simulink model "PMRAC_non_time_delay_final"  (R2022a)
settings: Solver=ode45  StartTime=0.0  StopTime=50  RelTol=1e-3  EnableMultiTasking=on
settings Model: Creator=Administrator  LastModifiedBy=mluser
settings SolverCC: AlgebraicLoopSolver=TrustRegion
settings DataIOCC: LimitDataPoints=on  SaveFormat=Array  ReturnWorkspaceOutputs=off
settings OptimizationCC: LifeSpan=inf
settings DebuggingCC: SolverPrmCheckMsg=warning  UnconnectedInputMsg=warning  UnconnectedOutputMsg=warning  UnconnectedLineMsg=warning  AllowSymbolicDim=off  SFUnexpectedBacktrackingDiag=warning  SFNoUnconditionalDefaultTransitionDiag=warning  SFExecutionAtInitializationDiag=none  SFMachineParentedDataDiag=warning  ArithmeticOperatorsInVariantConditions=warning
settings HardwareCC: ProdBitPerPointer=32  ProdBitPerSizeT=32  ProdBitPerPtrDiffT=32  ProdLargestAtomicFloat=None  ProdIntDivRoundTo=Undefined  ProdEndianess=Unspecified  ProdWordSize=32  ProdHWDeviceType=32-bit Generic
settings ModelReferenceCC: PropagateSignalLabelsOutOfModel=off
settings SFSimCC: SimUseLocalCustomCode=off  CustomCodeUndefinedFunction=UseInterfaceOnly
settings RTWCC: RTWUseLocalCustomCode=off
settings CodeAppCC: StateflowObjectComments=on
settings GRTTargetCC: TargetLangStandard=C89/C90 (ANSI)
settings ConfigComp: CovMetricSettings=dw  CovSaveCumulativeToWorkspaceVar=on  CovSaveSingleToWorkspaceVar=on  CovExternalEMLEnable=off  CovSFcnEnable=off

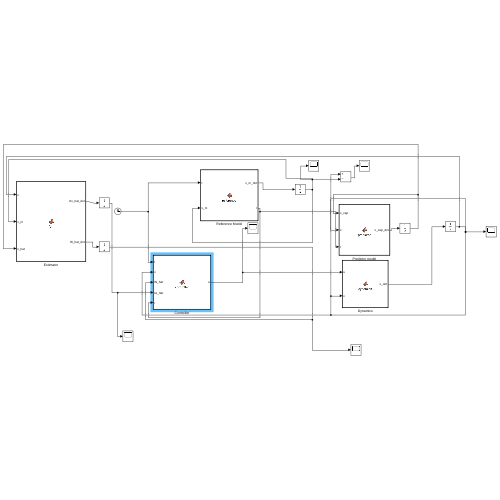
[thumbnail: Simulink's stored preview of the top-level diagram]
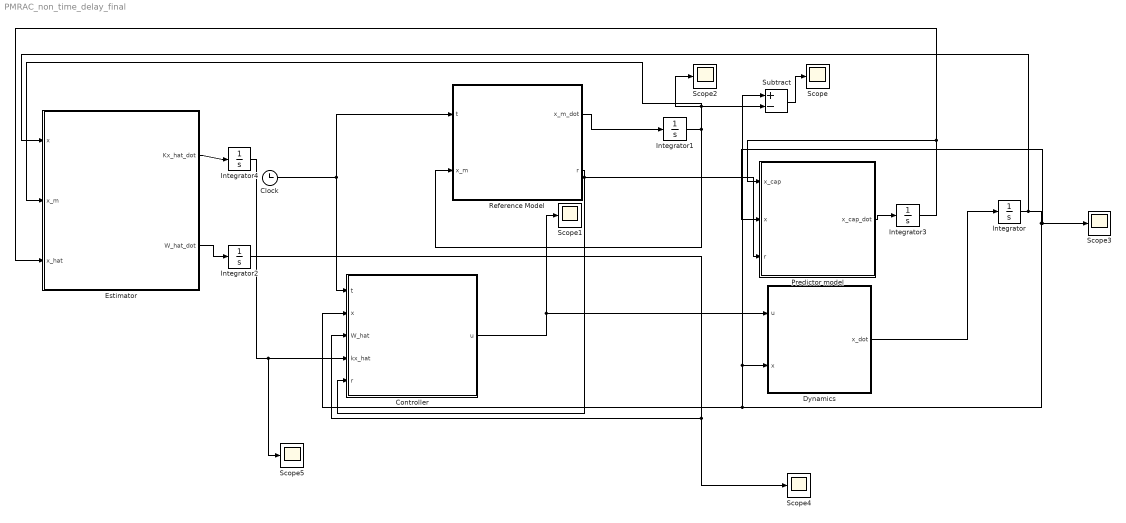
== system PMRAC_non_time_delay_final ==
  Clock : Clock
      settings: Decimation=50
  Controller : MATLAB Function  TreatAsAtomicUnit=on
  Dynamics : MATLAB Function  TreatAsAtomicUnit=on
  Estimator : MATLAB Function  TreatAsAtomicUnit=on
  Integrator : Integrator  InitialCondition=[-1;1]
  Integrator1 : Integrator  InitialCondition=[0;0]
  Integrator2 : Integrator  InitialCondition=zeros(6,1)
  Integrator3 : Integrator  InitialCondition=[-1;1]
  Integrator4 : Integrator  InitialCondition=zeros(2,1)
  Predictor model : MATLAB Function  TreatAsAtomicUnit=on
  Reference Model : MATLAB Function  TreatAsAtomicUnit=on
  Scope{,1..5} (6 alike) : Scope
  Subtract : Sum  Inputs=+-
  wires:
  Dynamics/1(x_dot) -> Integrator/1
  Integrator/1 -> Estimator/1(x), Predictor model/2(x), Scope3/1, Subtract/1, Dynamics/2(x), Controller/2(x)
  Clock/1 -> Controller/1(t), Reference Model/1(t)
  Controller/1(u) -> Scope1/1, Dynamics/1(u)
  Reference Model/1(x_m_dot) -> Integrator1/1
  Integrator1/1 -> Estimator/2(x_m), Subtract/2, Scope2/1, Reference Model/2(x_m)
  Integrator2/1 -> Scope4/1, Controller/3(W_hat)
  Subtract/1 -> Scope/1
  Predictor model/1(x_cap_dot) -> Integrator3/1
  Integrator3/1 -> Estimator/3(x_hat), Predictor model/1(x_cap)
  Estimator/2(W_hat_dot) -> Integrator2/1
  Estimator/1(Kx_hat_dot) -> Integrator4/1
  Integrator4/1 -> Scope5/1, Controller/4(kx_hat)
  Reference Model/2(r) -> Controller/5(r), Predictor model/3(r)

== matlab function PMRAC_non_time_delay_final/Controller ==
  data: u output; t input; x input; W_hat input; kx_hat input; r input
function u   = controller(t,x,W_hat,kx_hat,r)

%r=10;
%r=exp(-t);

%r=2*sin(t);

%k_x=[-2/3 -1/3]'; % note that the linear control gain is directly chosen instead of adapting with an assumption of $A$ matrix to be known
theta=x(1,1);
p=x(2,1);
phi_bar = [1; theta; p; abs(theta)*p; abs(p)*p; theta^3];

u=kx_hat'*x+r-W_hat'*phi_bar;

end

== matlab function PMRAC_non_time_delay_final/Dynamics ==
  data: u input; x input; x_dot output
function x_dot    = dynamics(u,x)

L_delta_a=1;

A=[0 1; 0 0];

a0=0.8;
a1=0.2314;
a2=0.6918;
a3=-0.6245;
a4=0.0095;
a5=0.0214;

B=[0 1]';

theta=x(1,1);
p=x(2,1);

%W = [a0;a1;a2;a3;a4;a5];
%phi_bar = [1; theta; p; abs(theta)*p; abs(p)*p; theta^3];
%phi_bar =[1;1;1;1;1;1];

delta=a0+a1*theta+a2*p+a3*abs(theta)*p+a4*abs(p)*p+a5*theta^3;
x_dot=A*x+B*(u+delta/L_delta_a);
end

== matlab function PMRAC_non_time_delay_final/Predictor model ==
  data: x_cap_dot output; x_cap input; x input; r input
function x_cap_dot = predictor( x_cap, x, r)


am1=-2;
am2=-1;
A_ref=[0 1; am1 am2];

A_prd =4* A_ref;


L_delta_a=1;
B_c=[0; L_delta_a];

x_cap_dot = A_prd*(x_cap-x) + A_ref*x + B_c*r;

== matlab function PMRAC_non_time_delay_final/Reference Model ==
  data: x_m_dot output; t input; x_m input; r output
function [x_m_dot,r]  = reference(t,x_m)
am1=-2;
am2=-1;
L_delta_a=1;
%r=exp(-t);
r=sin(t);
%r=2*sin(t);
%A_ref=A+B*k_x';
A_ref=[0 1; am1 am2];
B_c=[0; L_delta_a];
x_m_dot=A_ref*x_m+B_c*r;

== matlab function PMRAC_non_time_delay_final/Estimator ==
  data: Kx_hat_dot output; W_hat_dot output; x input; x_m input; x_hat input
function [Kx_hat_dot, W_hat_dot] = fcn(x, x_m, x_hat)

%gamma_x = [1,0;
 %          2,1];
gamma_x=2*eye(2);
%gamma_w = [1,0,1,2,3,4;
  %         3,4,1,2,5,6;
  %         5,2,1,6,8,3;
  %         2,4,5,7,2,1;
  %         4,5,1,2,6,3;
  %         7,9,0,1,3,0];
gamma_w=100*eye(6);

theta=x(1,1);
p=x(2,1);
phi_bar = [1; theta; p; abs(theta)*p; abs(p)*p; theta^3];

%P_ref = [1.75,-0.5;-0.5,3];
%P_ref=[3.5 0.5;0.5 1.5];
P_ref = [8.75,1.25;1.25,3.75];

P_prd =4* P_ref;
B=[0 1]';


Kx_hat_dot = -gamma_x*x*((x-x_m)'*P_ref-(x_hat-x)'*P_prd)*B;
W_hat_dot = gamma_w*phi_bar*((x-x_m)'*P_ref-(x_hat-x)'*P_prd)*B;
